simulink model "Model_Simscape"  (R2023a)
settings: Solver=VariableStepAuto  StartTime=0.0  StopTime=10.0  RelTol=1e-3
model workspace (MAT data in the model file):
  Air_density = 1.29
  Body_Temperature = 37
  CtrlData_Max = 100
  CtrlData_Min = 0
  Detpress_to_Vavle : object (value not decoded)
  E_respriatory = 10
  ExpValve : object (value not decoded)
  FRC = 2
  Fan : object (value not decoded)
  FanHousing : object (value not decoded)
  Flow_Resistance_1 : object (value not decoded)
  Flow_Resistance_2 : object (value not decoded)
  Hard_Stop : Lower_bound (value not decoded)
  InspValve : object (value not decoded)
  L_to_m3 = 0.001
  Mask : object (value not decoded)
  OxyValve : object (value not decoded)
  OxygenSensor : object (value not decoded)
  Pa_to_cmH2O = 0.0101974428892
  Percent_to_Unit = 0.01
  Pipe_1 : object (value not decoded)
  Pipe_2 : object (value not decoded)
  Pipe_3 : object (value not decoded)
  R_respiratory = 2
  Reservoir : Cross_area (value not decoded)
  Trachea : object (value not decoded)
  Volume_Max = 0.9
  cmH2O_to_Pa = 98.0638
  cmH2O_to_kPa = 0.0981
  lung : object (value not decoded)
  percentage_to_rpm = 600
symbols that are objects in the model workspace (value not decoded): ExpValve, FanHousing, Flow_Resistance_1, Flow_Resistance_2, InspValve, lung, OxygenSensor
libraries: fl_lib x81, nesl_utility x17, SimscapeFluids_lib x4, aerolibatmos2 x1
(part 4 of 4)

== system Model_Simscape/ExpValveModel/ Inlet Pressure Sensor ==
  Pressure & Temperature Sensor (G) : fl_lib/Gas/Sensors/Pressure & Temperature Sensor (G)  reference=foundation.enum.MeasurementReference.difference  pressure=true  pressure_spec=foundation.enum.PressureMeasementSpec.Absolute  temperature=false
      settings: InternalSimscapePortConfiguration="{\"Bottom\":[],\"Left\":[{\"id\":\"A\",\"label\":\"A\",\"type\":\"foundation.gas.gas\"}],\"Right\":[{\"id\":\"B\",\"label\":\"B\",\"type\":\"foundation.gas.gas\"},{\"id\":\"P\",\"label\":\"P\",\"type\":\"output\"}],\"Top\":[]}"
  Reservoir (G)1 : fl_lib/Gas/Elements/Reservoir (G)  pressure_spec=foundation.enum.pressure_spec.atmospheric  reservoir_pressure=0.101325 MPa  reservoir_temperature=293.15 K  area_A=Reservoir.Cross_area m^2
  A : PMIOPort  Side=Left
  InletPress : PMIOPort  Port=2  Side=Right
  connections:
  Reservoir (G)1/LConn1 -- Pressure & Temperature Sensor (G)/RConn1
  Pressure & Temperature Sensor (G)/RConn2 -- InletPress/RConn1
  Pressure & Temperature Sensor (G)/LConn1 -- A/RConn1

== system Model_Simscape/ExpValveModel/ Outlet Pressure Sensor ==
  Pressure & Temperature Sensor (G) : fl_lib/Gas/Sensors/Pressure & Temperature Sensor (G)  reference=foundation.enum.MeasurementReference.difference  pressure=true  pressure_spec=foundation.enum.PressureMeasementSpec.Absolute  temperature=false
      settings: InternalSimscapePortConfiguration="{\"Bottom\":[],\"Left\":[{\"id\":\"A\",\"label\":\"A\",\"type\":\"foundation.gas.gas\"}],\"Right\":[{\"id\":\"B\",\"label\":\"B\",\"type\":\"foundation.gas.gas\"},{\"id\":\"P\",\"label\":\"P\",\"type\":\"output\"}],\"Top\":[]}"
  Reservoir (G)1 : fl_lib/Gas/Elements/Reservoir (G)  pressure_spec=foundation.enum.pressure_spec.atmospheric  reservoir_pressure=0.101325 MPa  reservoir_temperature=293.15 K  area_A=Reservoir.Cross_area m^2
  A : PMIOPort  Side=Left
  OutletPress : PMIOPort  Port=2  Side=Right
  connections:
  Pressure & Temperature Sensor (G)/LConn1 -- A/RConn1
  Reservoir (G)1/LConn1 -- Pressure & Temperature Sensor (G)/RConn1
  OutletPress/RConn1 -- Pressure & Temperature Sensor (G)/RConn2

== system Model_Simscape/InspValveModel/ Inlet Pressure Sensor ==
  Pressure & Temperature Sensor (G) : fl_lib/Gas/Sensors/Pressure & Temperature Sensor (G)  reference=foundation.enum.MeasurementReference.difference  pressure=true  pressure_spec=foundation.enum.PressureMeasementSpec.Absolute  temperature=false
      settings: InternalSimscapePortConfiguration="{\"Bottom\":[],\"Left\":[{\"id\":\"A\",\"label\":\"A\",\"type\":\"foundation.gas.gas\"}],\"Right\":[{\"id\":\"B\",\"label\":\"B\",\"type\":\"foundation.gas.gas\"},{\"id\":\"P\",\"label\":\"P\",\"type\":\"output\"}],\"Top\":[]}"
  Reservoir (G)1 : fl_lib/Gas/Elements/Reservoir (G)  pressure_spec=foundation.enum.pressure_spec.atmospheric  reservoir_pressure=0.101325 MPa  reservoir_temperature=293.15 K  area_A=Reservoir.Cross_area m^2
  A : PMIOPort  Side=Left
  InletPress : PMIOPort  Port=2  Side=Right
  connections:
  Reservoir (G)1/LConn1 -- Pressure & Temperature Sensor (G)/RConn1
  Pressure & Temperature Sensor (G)/RConn2 -- InletPress/RConn1
  Pressure & Temperature Sensor (G)/LConn1 -- A/RConn1

== system Model_Simscape/InspValveModel/ Outlet Pressure Sensor ==
  Pressure & Temperature Sensor (G) : fl_lib/Gas/Sensors/Pressure & Temperature Sensor (G)  reference=foundation.enum.MeasurementReference.difference  pressure=true  pressure_spec=foundation.enum.PressureMeasementSpec.Absolute  temperature=false
      settings: InternalSimscapePortConfiguration="{\"Bottom\":[],\"Left\":[{\"id\":\"A\",\"label\":\"A\",\"type\":\"foundation.gas.gas\"}],\"Right\":[{\"id\":\"B\",\"label\":\"B\",\"type\":\"foundation.gas.gas\"},{\"id\":\"P\",\"label\":\"P\",\"type\":\"output\"}],\"Top\":[]}"
  Reservoir (G)1 : fl_lib/Gas/Elements/Reservoir (G)  pressure_spec=foundation.enum.pressure_spec.atmospheric  reservoir_pressure=0.101325 MPa  reservoir_temperature=293.15 K  area_A=Reservoir.Cross_area m^2
  A : PMIOPort  Side=Left
  OutletPress : PMIOPort  Port=2  Side=Right
  connections:
  Pressure & Temperature Sensor (G)/LConn1 -- A/RConn1
  Pressure & Temperature Sensor (G)/RConn2 -- OutletPress/RConn1
  Reservoir (G)1/LConn1 -- Pressure & Temperature Sensor (G)/RConn1

== system Model_Simscape/TurboModel/rpm to rad//s ==
  In1 : Inport  Unit=rpm
  Unit Conversion : UnitConversion
  Out1 : Outport  Unit=rad/s
  wires:
  Unit Conversion/1 -> Out1/1
  In1/1 -> Unit Conversion/1
